simulink model "controlled_rect"  (R2016a)
settings: Solver=ode4  StartTime=0.0  StopTime=2  FixedStep=1e-5  RelTol=1e-3
undefined symbols (not defined in the file): D1, lagging, pulse
libraries: powerlib_meascontrol x11, powerlib x10
settings Model: Creator=ugurm  LastModifiedBy=mesutto
settings DataIOCC: LimitDataPoints=on  SaveFormat=Array
settings DebuggingCC: UnderspecifiedInitializationDetection=Classic  MergeDetectMultiDrivingBlocksExec=none  SolverPrmCheckMsg=warning  StateNameClashWarn=warning
settings HardwareCC: ProdBitPerPointer=32  ProdLargestAtomicFloat=None  ProdIntDivRoundTo=Undefined  ProdEndianess=Unspecified  ProdWordSize=32  ProdHWDeviceType=32-bit Generic
settings ModelReferenceCC: PropagateSignalLabelsOutOfModel=off
settings ConfigComp: CovModelRefEnable=Off

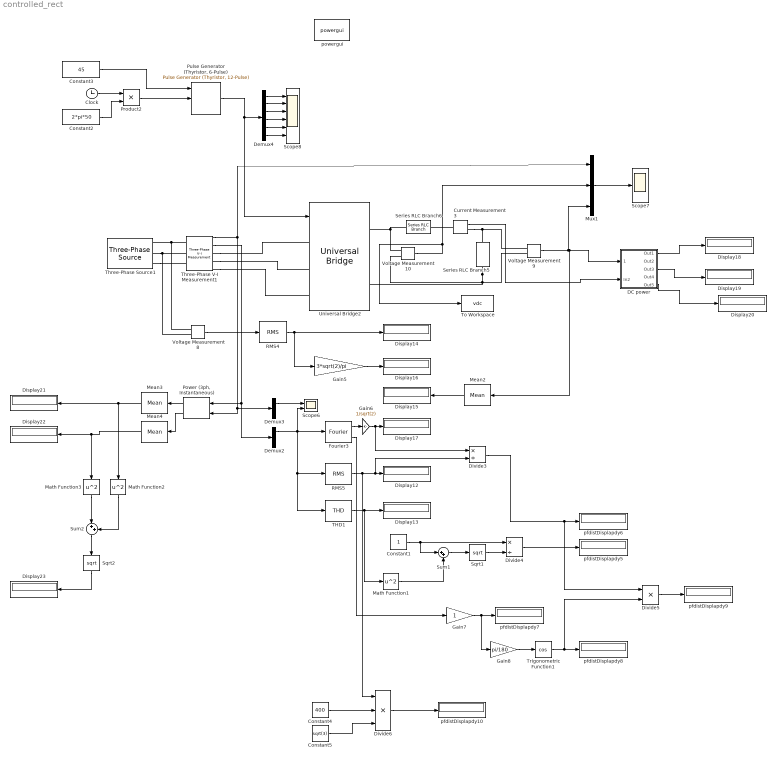
== system controlled_rect ==
  Clock : Clock
  Constant1 : Constant
  Constant2 : Constant  Value=2*pi*50
  Constant3 : Constant  Value=45
  Constant4 : Constant  Value=400
  Constant5 : Constant  Value=sqrt(3)
  Current Measurement3 : powerlib/Measurements/Current Measurement  PhasorSimulation=off  OutputType=Complex  PSBequivalent=0
  DC power : Subsystem
  Demux2 : Demux  Outputs=3
  Demux3 : Demux  Outputs=3
  Demux4 : Demux  Outputs=6
  Display{12..23} (12 alike) : Display
  Divide3 : Product  Inputs=*/
  Divide4 : Product  Inputs=*/
  Divide5 : Product  Inputs=**
  Divide6 : Product  Inputs=***
  Fourier3 : powerlib_meascontrol/Measurements/Fourier  Freq=50  n=1  InInit=[0, 0]  Ts=0
  Gain5 : Gain  Gain=3*sqrt(2)/pi
  Gain6 : Gain  Gain=1/sqrt(2)
  Gain7 : Gain
  Gain8 : Gain  Gain=pi/180
  Math Function1 : Math  Operator=square  SaturateOnIntegerOverflow=on
  Math Function2 : Math  Operator=square  SaturateOnIntegerOverflow=on
  Math Function3 : Math  Operator=square  SaturateOnIntegerOverflow=on
  Mean2 : powerlib_meascontrol/Measurements/Mean  Freq=50  Vinit=0  Ts=0
  Mean3 : powerlib_meascontrol/Measurements/Mean  Freq=50  Vinit=0  Ts=0
  Mean4 : powerlib_meascontrol/Measurements/Mean  Freq=50  Vinit=0  Ts=0
  Mux1 : Mux  Inputs=3
  "Power (3ph, Instantaneous)" : powerlib_meascontrol/Measurements/Power (3ph, Instantaneous)
  Product2 : Product
  "Pulse Generator (Thyristor, 6-Pulse)" : powerlib_meascontrol/Pulse & Signal Generators/Pulse Generator (Thyristor, 12-Pulse)  GenType=6-pulse  Delta=D1 (lagging)  pwidth=60  Double_Pulse=off  Ts=0
  RMS4 : powerlib_meascontrol/Measurements/RMS  TrueRMS=on  Freq=50  RMSInit=0  Ts=0
  RMS5 : powerlib_meascontrol/Measurements/RMS  TrueRMS=on  Freq=50  RMSInit=0  Ts=0
  Scope6 : Scope  NumInputPorts=2
  Scope7 : Scope
  Scope8 : Scope  NumInputPorts=6
  Series RLC Branch5 : powerlib/Elements/Series RLC Branch  LConnTagsString=__new0  RConnTagsString=__new0  BranchType=R  Resistance=5  Inductance=1/(2*pi*50)  SetiL0=off  InitialCurrent=0  Capacitance=1e-6  Setx0=off  InitialVoltage=0  Measurements=None
  Series RLC Branch6 : powerlib/Elements/Series RLC Branch  LConnTagsString=__new0  RConnTagsString=__new0  BranchType=L  Resistance=2  Inductance=100/(2*pi*50)  SetiL0=off  InitialCurrent=0  Capacitance=1e-6  Setx0=off  InitialVoltage=0  Measurements=None
  Sqrt1 : Sqrt  SaturateOnIntegerOverflow=on
  Sqrt2 : Sqrt  SaturateOnIntegerOverflow=on
  Sum1 : Sum  Inputs=|++
  Sum2 : Sum  Inputs=|++
  THD1 : powerlib_meascontrol/Measurements/THD  Freq=50  Ts=0
  Three-Phase V-I Measurement1 : powerlib/Measurements/Three-Phase V-I Measurement  VoltageMeasurement=phase-to-ground  SetLabelV=off  LabelV=Vabc  Vpu=off  VpuLL=off  CurrentMeasurement=yes  SetLabelI=off  LabelI=Iabc  Ipu=off  Pbase=100e6  Vbase=500e3  OutputType=Complex  PhasorSimulation=off  PSBequivalent=0
  Three-Phase Source1 : powerlib/Electrical Sources/Three-Phase Source  InternalConnection=Yg  VoltagePhases=off  Voltage=400  PhaseAngle=0  Voltage_phases=[25e3 25e3 25e3]/sqrt(3)  PhaseAngles_phases=[0 -120 +120]  Frequency=50  NonIdealSource=off  SpecifyImpedance=off  Resistance=0.8929  Inductance=16.58e-3  ShortCircuitLevel=100e6  BaseVoltage=25e3  XRratio=7  BusType=swing  Pref=10e3  Qref=0  Prefabc=[10e3, 10e3, 10e3]  Qrefabc=[0, 0, 0]  Qmin=-inf  Qmax=inf
  To Workspace : ToWorkspace  VariableName=vdc  SaveFormat=Structure With Time  SampleTime=-1
  Trigonometric Function1 : Trigonometry  Operator=cos
  Universal Bridge2 : powerlib/Power Electronics/Universal Bridge  Arms=3  SnubberResistance=1e5  SnubberCapacitance=inf  Device=Thyristors  Ron=1e-3  Lon=0  ForwardVoltages="[  0  0  ]"  ForwardVoltage=0  GTOparameters=[ 10e-6 , 20e-6 ]  IGBTparameters=[ 1e-6 , 2e-6 ]  Measurements=None  Measurements_2=None  converterType=Rectifier
  Voltage Measurement10 : powerlib/Measurements/Voltage Measurement  PhasorSimulation=off  OutputType=Complex  PSBequivalent=0
  Voltage Measurement8 : powerlib/Measurements/Voltage Measurement  PhasorSimulation=off  OutputType=Complex  PSBequivalent=0
  Voltage Measurement9 : powerlib/Measurements/Voltage Measurement  PhasorSimulation=off  OutputType=Complex  PSBequivalent=0
  pfdistDisplapdy{5..10} (6 alike) : Display
  powergui : powerlib/powergui  Priority=1  SimulationMode=Discrete  SolverType=Tustin/Backward Euler (TBE)  SampleTime=1e-5  frequency=60  SPID=off  DisableSnubberDevices=off  DisableRonSwitches=off  DisableVfSwitches=off  SwTol=0  DisplayEquations=off  Interpol=off  ExternalGateDelay=off  methode=off  Ts=10  FunctionMessages=off  echomessages=off  HookPort=off  EnableUseOfTLC=off  x0status=blocks  frequencyindice=50  Pbase=100e6  ErrMax=1e-4  Iterations=50  UnitsV=kV  UnitsW=MW  buscounter=0  RestoreLinks=warning  ResistiveCurrentMeasurement=off  Frange=[0:2:500]  Ylog=off  Xlog=on  ShowGrid=off  save=off  variable=ZData  structure=vdc  ZoomFFT=off  StartTime=0.2  cycles=20  DisplayStyle=5  fundamental=50  FreqAxis=off  MaxFrequency=2000  frequencyindicesteady=1  RmsSteady=1  display=off
  wires:
  Voltage Measurement9/1 -> Mux1/3, Mean2/1, DC power/1(voltage)
  RMS4/1 -> Gain5/1, Display14/1
  Mean2/1 -> Display15/1
  Gain5/1 -> Display16/1
  Three-Phase V-I Measurement1/1 -> "Power (3ph, Instantaneous)"/1, Demux3/1, Mux1/1
  Voltage Measurement10/1 -> To Workspace/1, Mux1/2
  Mux1/1 -> Scope7/1
  Voltage Measurement8/1 -> RMS4/1
  Three-Phase V-I Measurement1/2 -> Demux2/1, "Power (3ph, Instantaneous)"/2
  Demux2/1 -> THD1/1, RMS5/1, Scope6/2, Fourier3/1
  Fourier3/1 -> Gain6/1
  Current Measurement3/1 -> DC power/2(In2)
  Demux3/1 -> Scope6/1
  RMS5/1 -> Divide6/1, Divide3/2, Display12/1
  Gain6/1 -> Divide3/1, Display17/1
  THD1/1 -> Math Function1/1, Display13/1
  Divide3/1 -> Divide5/1, pfdistDisplapdy6/1
  Constant1/1 -> Sum1/1, Divide4/1
  Sqrt1/1 -> Divide4/2
  Math Function1/1 -> Sum1/2
  Sum1/1 -> Sqrt1/1
  Divide4/1 -> pfdistDisplapdy5/1
  Fourier3/2 -> Gain7/1
  Gain7/1 -> Gain8/1, pfdistDisplapdy7/1
  Trigonometric Function1/1 -> Divide5/2, pfdistDisplapdy8/1
  Divide5/1 -> pfdistDisplapdy9/1
  Gain8/1 -> Trigonometric Function1/1
  "Pulse Generator (Thyristor, 6-Pulse)"/1 -> Demux4/1, Universal Bridge2/1
  Product2/1 -> "Pulse Generator (Thyristor, 6-Pulse)"/2
  Clock/1 -> Product2/1
  Constant2/1 -> Product2/2
  Constant3/1 -> "Pulse Generator (Thyristor, 6-Pulse)"/1
  "Power (3ph, Instantaneous)"/2 -> Mean3/1
  "Power (3ph, Instantaneous)"/1 -> Mean4/1
  Mean3/1 -> Math Function2/1, Display21/1
  Mean4/1 -> Math Function3/1, Display22/1
  Constant5/1 -> Divide6/3
  Constant4/1 -> Divide6/2
  Math Function2/1 -> Sum2/2
  Math Function3/1 -> Sum2/1
  Sum2/1 -> Sqrt2/1
  Sqrt2/1 -> Display23/1
  Divide6/1 -> pfdistDisplapdy10/1
  Demux4/1 -> Scope8/1
  Demux4/3 -> Scope8/3
  Demux4/2 -> Scope8/2
  Demux4/4 -> Scope8/4
  Demux4/5 -> Scope8/5
  Demux4/6 -> Scope8/6
  DC power/1(Out1) -> Display18/1
  DC power/3(Out3) -> Display19/1
  DC power/5(Out5) -> Display20/1
  connections:
  Voltage Measurement9/LConn1 -- Current Measurement3/RConn1 -- Series RLC Branch5/LConn1
  Series RLC Branch5/RConn1 -- Voltage Measurement10/LConn2 -- Universal Bridge2/RConn2 -- Voltage Measurement9/LConn2
  Series RLC Branch6/RConn1 -- Voltage Measurement10/LConn1 -- Universal Bridge2/RConn1
  Three-Phase V-I Measurement1/LConn1 -- Voltage Measurement8/LConn1 -- Three-Phase Source1/RConn1
  Three-Phase Source1/RConn2 -- Voltage Measurement8/LConn2 -- Three-Phase V-I Measurement1/LConn2
  Three-Phase V-I Measurement1/RConn2 -- Universal Bridge2/LConn2
  Three-Phase V-I Measurement1/RConn1 -- Universal Bridge2/LConn1
  Current Measurement3/LConn1 -- Series RLC Branch6/LConn1
  Three-Phase Source1/RConn3 -- Three-Phase V-I Measurement1/LConn3
  Three-Phase V-I Measurement1/RConn3 -- Universal Bridge2/LConn3

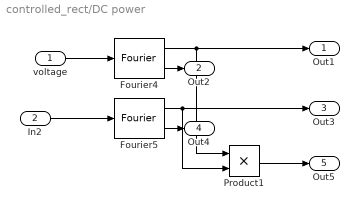
== system controlled_rect/DC power ==
  voltage : Inport
  In2 : Inport  Port=2
  Fourier4 : powerlib_meascontrol/Measurements/Fourier  Freq=50  n=0  InInit=[0, 0]  Ts=0
  Fourier5 : powerlib_meascontrol/Measurements/Fourier  Freq=50  n=0  InInit=[0, 0]  Ts=0
  Product1 : Product
  Out1 : Outport
  Out2 : Outport  Port=2
  Out3 : Outport  Port=3
  Out4 : Outport  Port=4
  Out5 : Outport  Port=5
  wires:
  Fourier4/2 -> Out2/1
  In2/1 -> Fourier5/1
  voltage/1 -> Fourier4/1
  Fourier5/2 -> Out4/1
  Product1/1 -> Out5/1
  Fourier5/1 -> Out3/1, Product1/2
  Fourier4/1 -> Out1/1, Product1/1
